simulink model "QBot2e_2D_Mapping_Manual"  (Simulink 8.9)
settings: Solver=ode1  StartTime=0.0  StopTime=inf  FixedStep=0.01  RelTol=1e-3  EnableMultiTasking=on
PreLoadFcn:
  | %open_system(find_system('Name', 'Video Viewer (MAP)'))
PostLoadFcn:
  | p=1:640; % pixels from left to right
  | 
  | Obtained_angles=(320-p).*(57/640)*pi./180;  % Kinect's horizontal FOV = 57 degrees
  | 
  | S=400;
  | 
  | %imageHandle = get_param(find_system('Name', 'Video Viewer (MAP)'), 'handle');
  | %ud = get_param(imageHandle{1}, 'UserData');
  | 
  | %figure_handle=ud.figure_handle;
  | %axes_handle = ud.axes_handle;
  | 
  | % set(figure_handle,'Position',[0 200 1000 800])
  | 
  | %ylim(axes_handle,[75 225]);
  | %xlim(axes_handle,[75 225]);
  | 
  | % open_system(find_system('Name', 'Video Viewer (MAP)'))
InitFcn:
  |  %open_system(find_system('Name', 'Display Image (MAP)'))
StartFcn:
  | %imageHandle = get_param(find_system('Name', 'Video Viewer (MAP)'), 'handle');
  | %ud = get_param(imageHandle{1}, 'UserData');
  | %axes_handle = ud.axes_handle;
  | 
  | %ylim(axes_handle,[75 225]);
  | %xlim(axes_handle,[75 225]);
undefined symbols (not defined in the file): HIL, qc_get_step_size, Video3D
libraries: quarc_library x9, simulink x2
settings Model: Creator=drmadill  LastModifiedBy=User  SimulationMode=external  ExtModeTrigDuration=2
settings SolverCC: PositivePriorityOrder=on  AutoInsertRateTranBlk=on
settings OptimizationCC: ExpressionDepthLimit=2147483647  LifeSpan=auto
settings DebuggingCC: SolverPrmCheckMsg=warning
settings RTWCC: SystemTargetFile=quarc_linux_pi_3.tlc  TemplateMakefile=quarc_linux_pi_3_tmf  Description=QUARC Linux Raspberry Pi 3 Target
settings STFCustomTargetCC: TargetLibSuffix=.a  TargetPreCompLibLocation=C:\PROGRA~3\QUARC\lib\2019b\LINUX_~1\release  ConcurrentExecutionCompliant=on  SystemTargetFile=quarc_linux_pi_3.tlc
settings GRTTargetCC: TargetLibSuffix=.a  TargetPreCompLibLocation=C:\PROGRA~3\QUARC\lib\2017a\LICFC8~1\release  ParMdlRefBuildCompliant=off  CompOptLevelCompliant=off  GeneratePreprocessorConditionals=Use local settings  MatFileLogging=off  CPPClassGenCompliant=off  UseToolchainInfoCompliant=off  ExtMode=on  ExtModeMexFile=quarc_comm  ExtModeMexArgs='-w -d /tmp -uri %u'
settings ConfigComp: CovSFcnEnable=off

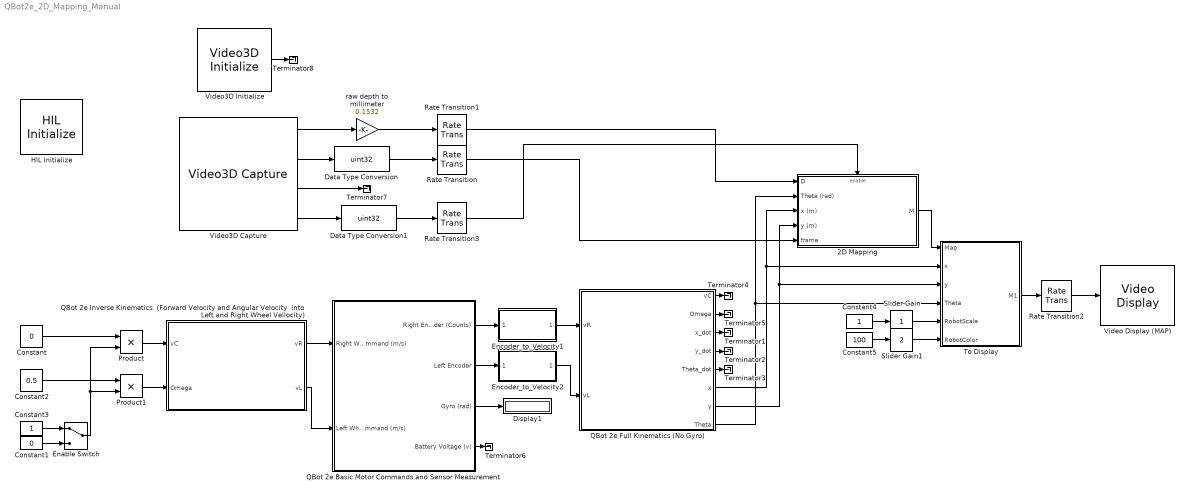
== system QBot2e_2D_Mapping_Manual ==
  2D Mapping : Subsystem  TreatAsAtomicUnit=on
  Constant : Constant  Value=0
  Constant1 : Constant  Value=0
  Constant2 : Constant  Value=0.5
  Constant3 : Constant
  Constant4 : Constant
  Constant5 : Constant  Value=100
  Data Type Conversion : DataTypeConversion  OutDataTypeStr=uint32
  Data Type Conversion1 : DataTypeConversion  OutDataTypeStr=uint32
  Display1 : Display
  Enable Switch : ManualSwitch
  Encoder_to_Velocity1 : Subsystem
  Encoder_to_Velocity2 : Subsystem
  HIL Initialize : quarc_library/Data Acquisition/Generic/Configuration/HIL Initialize  Priority=-99  object_name=HIL-1  board_type=qbot2e  board_number=0  board_options=pwm0_en=1;pwm0_pin=12;pwm1_en=1;pwm1_pin=13;  exclusive=off  active=off  hardware_clocks=[]  clock_modes=[]  initial_clock_frequencies=[]  set_clock_params_at_start=off  set_clock_params_at_switch_in=off  set_clock_frequencies_at_start=off  set_clock_frequencies_at_switch_in=off  analog_input_channels=[0:5]  analog_input_configurations=[]  analog_input_maximums=[16.5 3.3 3.3 3.3 3.3 3.3]  analog_input_minimums=[0 0 0 0 0 0]  set_analog_input_params_at_start=off  set_analog_input_params_at_switch_in=off  analog_output_channels=[]  analog_output_maximums=[]  analog_output_minimums=[]  initial_analog_outputs=[]  final_analog_outputs=[]  watchdog_analog_outputs=[]  set_analog_output_params_at_start=off  set_analog_output_params_at_switch_in=off  set_analog_outputs_at_start=off  set_analog_outputs_at_switch_in=off  set_analog_outputs_at_terminate=off  set_analog_outputs_at_switch_out=off  set_analog_outputs_on_watchdog=off  digital_input_channels=[28:58]  digital_output_channels=[28:31]  digital_output_configuration=[]  initial_digital_outputs=[0]  final_digital_outputs=[0]  watchdog_digital_outputs=[]  set_digital_output_params_at_start=off  set_digital_output_params_at_switch_in=off  set_digital_outputs_at_start=on  set_digital_outputs_at_switch_in=off  set_digital_outputs_at_terminate=on  set_digital_outputs_at_switch_out=off  set_digital_outputs_on_watchdog=off  encoder_channels=[0:1]  quadrature=[4]  encoder_filter_frequency=[]  initial_encoder_counts=[0]  set_encoder_params_at_start=on  set_encoder_params_at_switch_in=off  set_encoder_counts_at_start=on  set_encoder_counts_at_switch_in=off  pwm_channels=[0:1]  pwm_modes=0  pwm_frequency=100e6 / 4095  pwm_configuration=[0]  pwm_alignment=[0]  pwm_polarity=[1]  pwm_leading_deadband=[]  pwm_trailing_deadband=[]  initial_pwm_outputs=[0]  final_pwm_outputs=[0]  watchdog_pwm_outputs=[]  set_pwm_params_at_start=on  set_pwm_params_at_switch_in=off  set_pwm_outputs_at_start=on  set_pwm_outputs_at_switch_in=off  set_pwm_outputs_at_terminate=on  set_pwm_outputs_at_switch_out=off  set_pwm_outputs_on_watchdog=off  other_output_channels=[2000:2001 14000 16000]  initial_other_outputs=[0 0 0 7]  final_other_outputs=[0 0 0 7]  watchdog_other_outputs=[]  set_other_outputs_at_start=on  set_other_outputs_at_switch_in=off  set_other_outputs_at_terminate=on  set_other_outputs_at_switch_out=off  set_other_outputs_on_watchdog=off
  Product : Product  RndMeth=Zero
  Product1 : Product  RndMeth=Zero
  QBot 2e Basic Motor Commands and Sensor Measurement : Subsystem
  QBot 2e Full Kinematics (No Gyro) : Subsystem
  QBot 2e Inverse Kinematics  (Forward Velocity and Angular Velocity  into Left and Right Wheel Vellocity) : Subsystem
  Rate Transition : RateTransition  X0=uint32(0)
  Rate Transition1 : RateTransition
  Rate Transition2 : RateTransition
  Rate Transition3 : RateTransition
  Slider Gain : simulink/Math Operations/Slider Gain  gain=1  low=0  high=10
  Slider Gain1 : simulink/Math Operations/Slider Gain  gain=2  low=0.5  high=2.5
  Terminator{1..8} (8 alike) : Terminator
  To Display : MATLAB Function  TreatAsAtomicUnit=on
  Video Display (MAP) : quarc_library/Multimedia/Video Display  Tag=QBot2e_2D_Mapping_Manual/Video Display (MAP)  sample_time=-1  use_hardware=on
  Video3D Capture : quarc_library/Multimedia/Video3D Capture  object_name=Video3D-1  stream_type=Depth  stream_index=0  resolution=640 x 480  width=640  height=480  output_format=MATLAB greyscale (HxW)  data_type=uint16  sample_time=qc_get_step_size * ceil(0.033 / qc_get_step_size)  brightness_override=off  brightness=50.0  contrast_override=off  contrast=50.0  hue_override=off  hue=50.0  saturation_override=off  saturation=50.0  sharpness_override=off  sharpness=50.0  gamma_override=off  gamma=50.0  gain_override=off  gain=50.0  backlightcompensation_override=off  backlightcompensation=50.0  whitebalance_override=Automatic white balance  whitebalance=50.0  exposure_override=Automatic exposure  exposure=30.0  emitter=Enable laser emitter  preset=Do not set camera presets
  Video3D Initialize : quarc_library/Multimedia/Video3D Initialize  object_name=Video3D-1  source=Device  identifier=0  file=sample.bag  sample_time=qc_get_step_size * ceil(0.033 / qc_get_step_size)  active=on
  raw depth to millimeter : Gain  Gain=0.1532
  wires:
  Constant3/1 -> Enable Switch/1
  Constant1/1 -> Enable Switch/2
  QBot 2e Basic Motor Commands and Sensor Measurement/1(Right Encoder (Counts)) -> Encoder_to_Velocity1/1(Encoder)
  QBot 2e Basic Motor Commands and Sensor Measurement/2(Left Encoder) -> Encoder_to_Velocity2/1(Encoder)
  QBot 2e Basic Motor Commands and Sensor Measurement/3(Gyro (rad)) -> Display1/1
  QBot 2e Full Kinematics (No Gyro)/8(Theta) -> 2D Mapping/2(Theta (rad)), To Display/4(Theta)
  QBot 2e Full Kinematics (No Gyro)/7(y) -> 2D Mapping/4(y (m)), To Display/3(y)
  QBot 2e Full Kinematics (No Gyro)/6(x) -> 2D Mapping/3(x (m)), To Display/2(x)
  Encoder_to_Velocity1/1(Velocity) -> QBot 2e Full Kinematics (No Gyro)/1(vR)
  Encoder_to_Velocity2/1(Velocity) -> QBot 2e Full Kinematics (No Gyro)/2(vL)
  Constant/1 -> Product/1
  Constant2/1 -> Product1/1
  QBot 2e Inverse Kinematics  (Forward Velocity and Angular Velocity  into Left and Right Wheel Vellocity)/1(vR) -> QBot 2e Basic Motor Commands and Sensor Measurement/1(Right Wheel Command (m/s))
  QBot 2e Inverse Kinematics  (Forward Velocity and Angular Velocity  into Left and Right Wheel Vellocity)/2(vL) -> QBot 2e Basic Motor Commands and Sensor Measurement/2(Left Wheel Command (m/s))
  Product/1 -> QBot 2e Inverse Kinematics  (Forward Velocity and Angular Velocity  into Left and Right Wheel Vellocity)/1(vC)
  Product1/1 -> QBot 2e Inverse Kinematics  (Forward Velocity and Angular Velocity  into Left and Right Wheel Vellocity)/2(Omega)
  Enable Switch/1 -> Product/2, Product1/2
  2D Mapping/1(M) -> To Display/1(Map)
  To Display/1(M1) -> Rate Transition2/1
  Constant4/1 -> Slider Gain/1
  Slider Gain/1 -> To Display/5(RobotScale)
  Constant5/1 -> Slider Gain1/1
  Slider Gain1/1 -> To Display/6(RobotColor)
  QBot 2e Full Kinematics (No Gyro)/3(x_dot) -> Terminator1/1
  QBot 2e Full Kinematics (No Gyro)/4(y_dot) -> Terminator2/1
  QBot 2e Full Kinematics (No Gyro)/5(Theta_dot) -> Terminator3/1
  QBot 2e Full Kinematics (No Gyro)/1(vC) -> Terminator4/1
  QBot 2e Full Kinematics (No Gyro)/2(Omega) -> Terminator5/1
  Rate Transition2/1 -> Video Display (MAP)/1
  QBot 2e Basic Motor Commands and Sensor Measurement/4(Battery Voltage (v)) -> Terminator6/1
  Video3D Initialize/1 -> Terminator8/1
  Video3D Capture/2 -> Data Type Conversion/1
  Video3D Capture/1 -> raw depth to millimeter/1
  Rate Transition1/1 -> 2D Mapping/1(D)
  Video3D Capture/3 -> Terminator7/1
  Video3D Capture/4 -> Data Type Conversion1/1
  Data Type Conversion/1 -> Rate Transition/1
  Rate Transition3/1 -> 2D Mapping/Enable
  Rate Transition/1 -> 2D Mapping/5(frame)
  Data Type Conversion1/1 -> Rate Transition3/1
  raw depth to millimeter/1 -> Rate Transition1/1

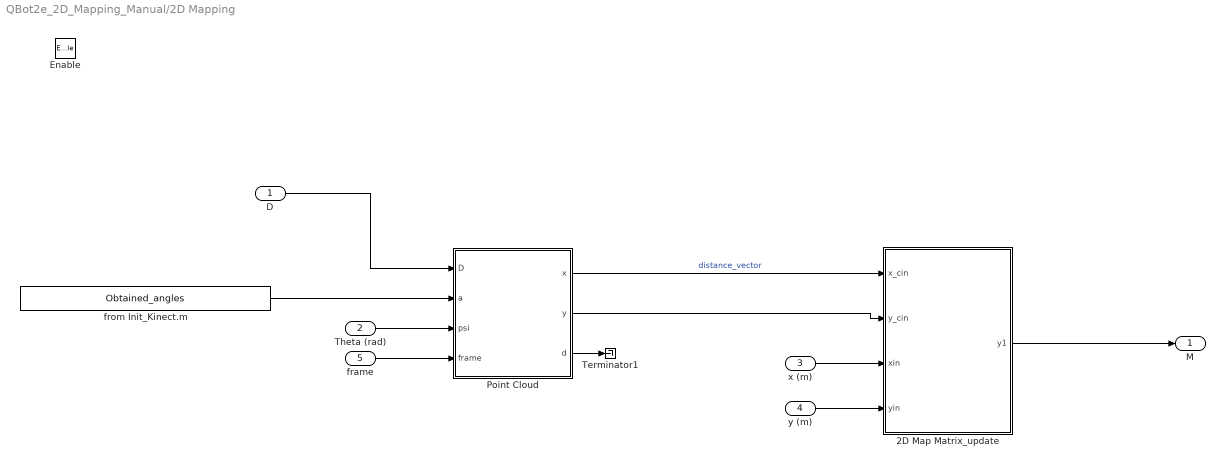
== system QBot2e_2D_Mapping_Manual/2D Mapping ==
  D : Inport
  Theta (rad) : Inport  Port=2
  x (m) : Inport  Port=3
  y (m) : Inport  Port=4
  frame : Inport  Port=5
  Enable : EnablePort
  2D Map Matrix_update : MATLAB Function  TreatAsAtomicUnit=on
  Point Cloud : MATLAB Function  TreatAsAtomicUnit=on
  Terminator1 : Terminator
  from Init_Kinect.m : Constant  Value=Obtained_angles
  M : Outport
  wires:
  from Init_Kinect.m/1 -> Point Cloud/2(a)
  Point Cloud/1(x) -> 2D Map Matrix_update/1(x_cin)  "distance_vector"
  Point Cloud/2(y) -> 2D Map Matrix_update/2(y_cin)
  Point Cloud/3(d) -> Terminator1/1
  D/1 -> Point Cloud/1(D)
  2D Map Matrix_update/1(y1) -> M/1
  Theta (rad)/1 -> Point Cloud/3(psi)
  x (m)/1 -> 2D Map Matrix_update/3(xin)
  y (m)/1 -> 2D Map Matrix_update/4(yin)
  frame/1 -> Point Cloud/4(frame)

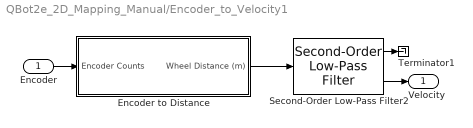
== system QBot2e_2D_Mapping_Manual/Encoder_to_Velocity1 ==
  Encoder : Inport
  Encoder to Distance : Subsystem
  Second-Order Low-Pass Filter2 : quarc_library/Continuous/Second-Order Low-Pass Filter  params_source=Internal (dialog parameters)  input_width=10  input_zeta=1  input_init=0
  Terminator1 : Terminator
  Velocity : Outport
  wires:
  Second-Order Low-Pass Filter2/1 -> Terminator1/1
  Encoder to Distance/1(Wheel Distance (m)) -> Second-Order Low-Pass Filter2/1
  Encoder/1 -> Encoder to Distance/1(Encoder Counts)
  Second-Order Low-Pass Filter2/2 -> Velocity/1

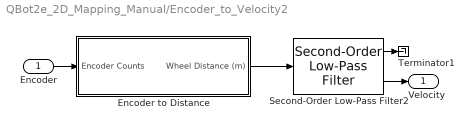
== system QBot2e_2D_Mapping_Manual/Encoder_to_Velocity2 ==
  Encoder : Inport
  Encoder to Distance : Subsystem
  Second-Order Low-Pass Filter2 : quarc_library/Continuous/Second-Order Low-Pass Filter  params_source=Internal (dialog parameters)  input_width=10  input_zeta=1  input_init=0
  Terminator1 : Terminator
  Velocity : Outport
  wires:
  Second-Order Low-Pass Filter2/2 -> Velocity/1
  Encoder/1 -> Encoder to Distance/1(Encoder Counts)
  Encoder to Distance/1(Wheel Distance (m)) -> Second-Order Low-Pass Filter2/1
  Second-Order Low-Pass Filter2/1 -> Terminator1/1

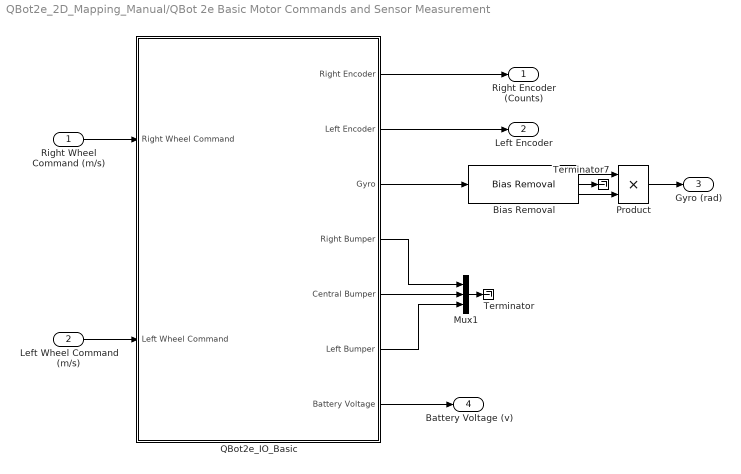
== system QBot2e_2D_Mapping_Manual/QBot 2e Basic Motor Commands and Sensor Measurement ==
  Right Wheel Command (m/s) : Inport
  Left Wheel Command (m/s) : Inport  Port=2
  Bias Removal : quarc_library/Discrete/Bias Removal  start_time=3  end_time=4  switch_id=0  sample_time=qc_get_step_size
      settings: SourceProductName=QUARC Targets
  Mux1 : Mux  Inputs=3
  Product : Product  RndMeth=Zero
  QBot2e_IO_Basic : Subsystem
  Terminator : Terminator
  Terminator7 : Terminator
  Right Encoder (Counts) : Outport
  Left Encoder : Outport  Port=2
  Gyro (rad) : Outport  Port=3
  Battery Voltage (v) : Outport  Port=4
  wires:
  QBot2e_IO_Basic/4(Right Bumper) -> Mux1/1
  QBot2e_IO_Basic/5(Central Bumper) -> Mux1/2
  QBot2e_IO_Basic/6(Left Bumper) -> Mux1/3
  Right Wheel Command (m/s)/1 -> QBot2e_IO_Basic/1(Right Wheel Command)
  Left Wheel Command (m/s)/1 -> QBot2e_IO_Basic/2(Left Wheel Command)
  QBot2e_IO_Basic/1(Right Encoder) -> Right Encoder (Counts)/1
  QBot2e_IO_Basic/2(Left Encoder) -> Left Encoder/1
  QBot2e_IO_Basic/7(Battery Voltage) -> Battery Voltage (v)/1
  Bias Removal/2 -> Terminator7/1
  Bias Removal/1 -> Product/1
  Bias Removal/3 -> Product/2
  Product/1 -> Gyro (rad)/1
  QBot2e_IO_Basic/3(Gyro) -> Bias Removal/1
  Mux1/1 -> Terminator/1

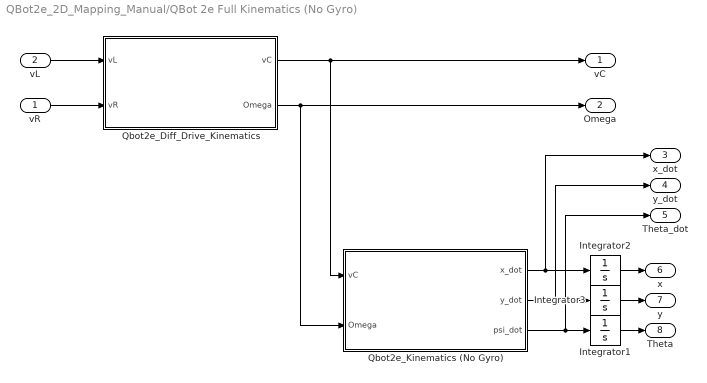
== system QBot2e_2D_Mapping_Manual/QBot 2e Full Kinematics (No Gyro) ==
  vR : Inport
  vL : Inport  Port=2
  Integrator1 : Integrator
  Integrator2 : Integrator
  Integrator3 : Integrator
  Qbot2e_Diff_Drive_Kinematics : Subsystem
  Qbot2e_Kinematics (No Gyro) : Subsystem
  vC : Outport
  Omega : Outport  Port=2
  x_dot : Outport  Port=3
  y_dot : Outport  Port=4
  Theta_dot : Outport  Port=5
  x : Outport  Port=6
  y : Outport  Port=7
  Theta : Outport  Port=8
  wires:
  Integrator1/1 -> Theta/1
  Qbot2e_Kinematics (No Gyro)/3(psi_dot) -> Theta_dot/1, Integrator1/1
  Qbot2e_Kinematics (No Gyro)/1(x_dot) -> x_dot/1, Integrator2/1
  Qbot2e_Kinematics (No Gyro)/2(y_dot) -> y_dot/1, Integrator3/1
  Qbot2e_Diff_Drive_Kinematics/1(vC) -> Qbot2e_Kinematics (No Gyro)/1(vC), vC/1
  vL/1 -> Qbot2e_Diff_Drive_Kinematics/1(vL)
  vR/1 -> Qbot2e_Diff_Drive_Kinematics/2(vR)
  Integrator2/1 -> x/1
  Integrator3/1 -> y/1
  Qbot2e_Diff_Drive_Kinematics/2(Omega) -> Qbot2e_Kinematics (No Gyro)/2(Omega), Omega/1

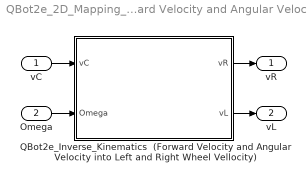
== system QBot2e_2D_Mapping_Manual/QBot 2e Inverse Kinematics  (Forward Velocity and Angular Velocity  into Left and Right Wheel Vellocity) ==
  vC : Inport
  Omega : Inport  Port=2
  QBot2e_Inverse_Kinematics  (Forward Velocity and Angular Velocity into Left and Right Wheel Vellocity) : MATLAB Function  TreatAsAtomicUnit=on
  vR : Outport
  vL : Outport  Port=2
  wires:
  QBot2e_Inverse_Kinematics  (Forward Velocity and Angular Velocity into Left and Right Wheel Vellocity)/2(vL) -> vL/1
  Omega/1 -> QBot2e_Inverse_Kinematics  (Forward Velocity and Angular Velocity into Left and Right Wheel Vellocity)/2(Omega)
  QBot2e_Inverse_Kinematics  (Forward Velocity and Angular Velocity into Left and Right Wheel Vellocity)/1(vR) -> vR/1
  vC/1 -> QBot2e_Inverse_Kinematics  (Forward Velocity and Angular Velocity into Left and Right Wheel Vellocity)/1(vC)

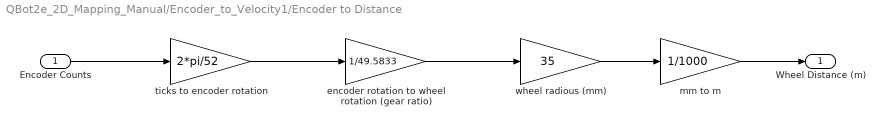
== system QBot2e_2D_Mapping_Manual/Encoder_to_Velocity1/Encoder to Distance ==
  Encoder Counts : Inport
  " encoder rotation to wheel rotation (gear ratio)" : Gain  Gain=1/49.5833
  mm to m : Gain  Gain=1/1000
  ticks to encoder rotation : Gain  Gain=2*pi/52
  wheel radious (mm) : Gain  Gain=35
  Wheel Distance (m) : Outport
  wires:
  Encoder Counts/1 -> ticks to encoder rotation/1
  ticks to encoder rotation/1 -> " encoder rotation to wheel rotation (gear ratio)"/1
  " encoder rotation to wheel rotation (gear ratio)"/1 -> wheel radious (mm)/1
  wheel radious (mm)/1 -> mm to m/1
  mm to m/1 -> Wheel Distance (m)/1

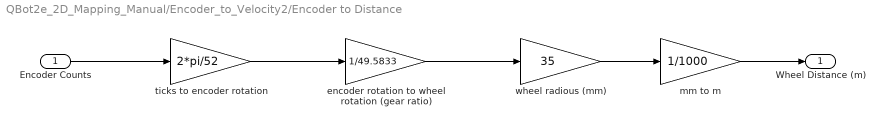
== system QBot2e_2D_Mapping_Manual/Encoder_to_Velocity2/Encoder to Distance ==
  Encoder Counts : Inport
  " encoder rotation to wheel rotation (gear ratio)" : Gain  Gain=1/49.5833
  mm to m : Gain  Gain=1/1000
  ticks to encoder rotation : Gain  Gain=2*pi/52
  wheel radious (mm) : Gain  Gain=35
  Wheel Distance (m) : Outport
  wires:
  mm to m/1 -> Wheel Distance (m)/1
  wheel radious (mm)/1 -> mm to m/1
  " encoder rotation to wheel rotation (gear ratio)"/1 -> wheel radious (mm)/1
  ticks to encoder rotation/1 -> " encoder rotation to wheel rotation (gear ratio)"/1
  Encoder Counts/1 -> ticks to encoder rotation/1

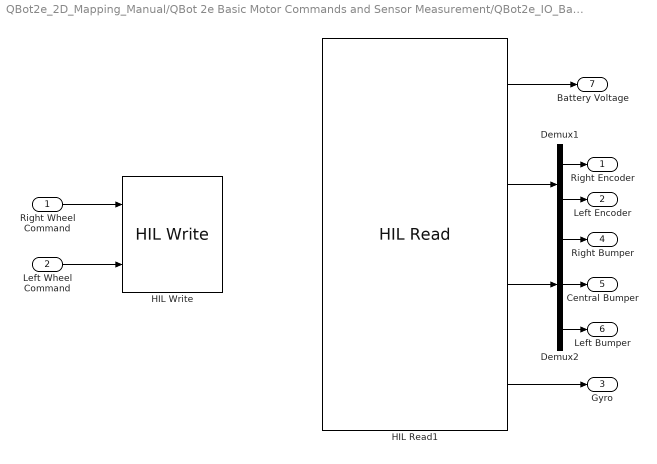
== system QBot2e_2D_Mapping_Manual/QBot 2e Basic Motor Commands and Sensor Measurement/QBot2e_IO_Basic ==
  Right Wheel Command : Inport
  Left Wheel Command : Inport  Port=2
  Demux1 : Demux  Outputs=2
  Demux2 : Demux  Outputs=3
  HIL Read1 : quarc_library/Data Acquisition/Generic/Immediate I//O/HIL Read  object_name=HIL-1  analog_channels=[0]  encoder_channels=[0:1]  digital_channels=[28:30]  other_channels=[1002]  sample_time=qc_get_step_size  active=on  vector_output=on  data_type_mode=Inherit via back propagation  encoder_data_type=double  digital_data_type=boolean
  HIL Write : quarc_library/Data Acquisition/Generic/Immediate I//O/HIL Write  object_name=HIL-1  analog_channels=[]  pwm_channels=[]  digital_channels=[]  other_channels=[2000:2001]  sample_time=-1  active=on  vector_input=off
  Right Encoder : Outport
  Left Encoder : Outport  Port=2
  Gyro : Outport  Port=3
  Right Bumper : Outport  Port=4
  Central Bumper : Outport  Port=5
  Left Bumper : Outport  Port=6
  Battery Voltage : Outport  Port=7
  wires:
  HIL Read1/1 -> Battery Voltage/1
  HIL Read1/3 -> Demux2/1
  HIL Read1/4 -> Gyro/1
  Demux1/1 -> Right Encoder/1
  Demux1/2 -> Left Encoder/1
  Right Wheel Command/1 -> HIL Write/1
  Left Wheel Command/1 -> HIL Write/2
  HIL Read1/2 -> Demux1/1
  Demux2/1 -> Right Bumper/1
  Demux2/2 -> Central Bumper/1
  Demux2/3 -> Left Bumper/1

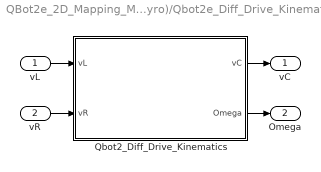
== system QBot2e_2D_Mapping_Manual/QBot 2e Full Kinematics (No Gyro)/Qbot2e_Diff_Drive_Kinematics ==
  vL : Inport
  vR : Inport  Port=2
  Qbot2_Diff_Drive_Kinematics : MATLAB Function  TreatAsAtomicUnit=on
  vC : Outport
  Omega : Outport  Port=2
  wires:
  vL/1 -> Qbot2_Diff_Drive_Kinematics/1(vL)
  Qbot2_Diff_Drive_Kinematics/1(vC) -> vC/1
  vR/1 -> Qbot2_Diff_Drive_Kinematics/2(vR)
  Qbot2_Diff_Drive_Kinematics/2(Omega) -> Omega/1

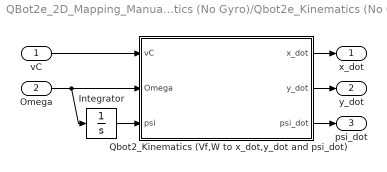
== system QBot2e_2D_Mapping_Manual/QBot 2e Full Kinematics (No Gyro)/Qbot2e_Kinematics (No Gyro) ==
  vC : Inport
  Omega : Inport  Port=2
  Integrator : Integrator
  Qbot2_Kinematics (Vf,W to x_dot,y_dot and psi_dot) : MATLAB Function  TreatAsAtomicUnit=on
  x_dot : Outport
  y_dot : Outport  Port=2
  psi_dot : Outport  Port=3
  wires:
  Qbot2_Kinematics (Vf,W to x_dot,y_dot and psi_dot)/3(psi_dot) -> psi_dot/1
  Integrator/1 -> Qbot2_Kinematics (Vf,W to x_dot,y_dot and psi_dot)/3(psi)
  vC/1 -> Qbot2_Kinematics (Vf,W to x_dot,y_dot and psi_dot)/1(vC)
  Qbot2_Kinematics (Vf,W to x_dot,y_dot and psi_dot)/1(x_dot) -> x_dot/1
  Omega/1 -> Integrator/1, Qbot2_Kinematics (Vf,W to x_dot,y_dot and psi_dot)/2(Omega)
  Qbot2_Kinematics (Vf,W to x_dot,y_dot and psi_dot)/2(y_dot) -> y_dot/1

== matlab function 2D Mapping/Point Cloud ==
  settings: sampleTime=qc_get_step_size
  data: D input double; x output double; y output double; a input double; psi input double; d output double; frame input double
function [x, y, d]  = fcn(D,a,psi,frame)
%#codegen


 %psi = psi; 
 a = -a; 
  
    LINE=240;

    x=zeros(1,640);
    y=zeros(1,640);

    r=double(D(LINE,:))';
    %d=0.1236*tan((r/2842.5)+1.1863);
    d=r/1000;

    d(d<0.5) = 0;
   
    
    
%d((d<0.5)==1)=0;


    L=d./cos(a);

    
    % robust check for max range
    if (frame>5) && sum(d)>0
        for i=15:625
            c=0;
            for j=-14:14
                if (L(i+j)==0)
                    c=c+1;
                end
            end
            if c>28
                L(i)=5.5;
            end
        end
    end
    
    x_r=L.*(cos(-a));
    y_r=L.*(sin(-a));
        

   
    
    R=[cos(psi) -sin(psi)
    sin(psi) cos(psi)];

   
    for j=1:640
        XY=R*[x_r(j);y_r(j)];
        x(j)=XY(1);
        y(j)=XY(2);
    end

    
  %alpha= -(LINE-240)*43*pi/180/480; % Vertical FOV
  %z=  tan(alpha)*L.*ones(640,1);

== matlab function QBot 2e Full Kinematics (No Gyro)/Qbot2e_Diff_Drive_Kinematics/Qbot2_Diff_Drive_Kinematics ==
  data: vL input double; vC output double; vR input double; Omega output double
function [vC,Omega] = fcn(vL,vR)
%#codegen

d= 0.235;

vC=0.5*(vL+vR);
Omega=(1/d)*(vR-vL);

== matlab function QBot 2e Full Kinematics (No Gyro)/Qbot2e_Kinematics (No Gyro)/Qbot2_Kinematics (Vf,W to x_dot,y_dot and psi_dot) ==
  data: vC input double; x_dot output double; Omega input double; y_dot output double; psi input double; psi_dot output double
function [x_dot,y_dot,psi_dot] = fcn(vC,Omega,psi)
%#codegen


x_dot=cos(psi)*vC;
y_dot=sin(psi)*vC;
psi_dot= Omega;

== matlab function To Display ==
  data: Map input double; x input double; y input double; Theta input double; M1 output double; RobotScale input double; RobotColor input double
function M1 = fcn(Map,x,y,Theta,RobotScale, RobotColor)
%#codegen
S=300;
scale=S/30;

r = 2*RobotScale+1; % magnitude (length) of arrow to plot

for i=1:r
        Uri=round(i*cos(Theta));
        Vri=round(i*sin(Theta));
        j=-(r-1)/2+i-1;
        Uli=round(j*cos(Theta-pi/2));
        Vli=round(j*sin(Theta-pi/2));
        Map(S/2+round(x*scale)+1+Uri,S/2+round(y*scale)+1+Vri)=RobotColor;  
        Map(S/2+round(x*scale)+1+Uli,S/2+round(y*scale)+1+Vli)=RobotColor;
end

% drawing the circle
for t=0:0.1:2*pi
        Xri=round(r*cos(t));
        Yri=round(r*sin(t));
        Map(S/2+round(x*scale)+1+Xri,S/2+round(y*scale)+1+Yri)=RobotColor;  
end


M1=Map;

== matlab function 2D Mapping/2D Map Matrix_update ==
  settings: updateMethod=DISCRETE  sampleTime=qc_get_step_size
  data: x_cin input double; y_cin input double; xin input double; yin input double; y1 output double
function y1 = fcn(x_cin,y_cin,xin, yin)
%#codegen

S=300;
scale=S/30;


x = round(xin*scale);
y = round(yin*scale);

x_c = round(x_cin*scale+x);
y_c = round(y_cin*scale+y);

%z_c = round(x_c*scale+0);

persistent M;

if isempty(M)
    M=uint8(100*ones(S+1,S+1));
end



    for i=1:length(x_c)

        if (sqrt((x_c(i)-x)^2+(y_c(i)-y)^2))/scale<=5.40 % add information only when data is within the valid range 
            M((x_c(i)+S/2+1),(y_c(i)+S/2+1))=0; % matrix indices start from 1 + centre the data
        end

        
        % refreshing the old data within the FOV cone
        Dist_Lx= (x_c(i)-x);
        Dist_Ly=(y_c(i)-y);
        L=[Dist_Lx,Dist_Ly];


        [m, m_idx] = max([abs(L(1)), abs(L(2))]);

        if m>0
            if m_idx(1)==1 % diff in x is larger
                for k=0: sign(L(1)): x_c(i)-x - sign(L(1))
                    M(x+S/2+k+1,y+round(Dist_Ly*k/Dist_Lx)+S/2+1)=255;
                end
            end

            if m_idx(1)==2
                for k=0: sign(L(2)): y_c(i)-y - sign(L(2))
                    M(x+round(Dist_Lx*k/Dist_Ly)+S/2+1,y+k+S/2+1)=255;
                end
            end
        end
        
        


    end



y1=M;

== matlab function QBot 2e Inverse Kinematics (Forward Velocity and Angular Velocity into Left and Right Wheel Vellocity)/QBot2e_Inverse_Kinematics (Forward Velocity and Angular Velocity into Left and Right Wheel Vellocity) ==
  data: vR output double; vL output double; vC input double; Omega input double
function [vR,vL] = fcn(vC , Omega)
%#codegen

d=0.235; 
% Eqn Based on the eqn 4.52 (W is the angular velocity)

vR = vC + Omega*d/2;
vL= vC - Omega*d/2;
